simulink model "Assignment_5"  (R2025b)
settings: Solver=FixedStepAuto  StartTime=0.0  StopTime=100  FixedStep=0.05  RelTol=1e-3
settings Model: PacingRate=10  Creator=ArriGE66  LastModifiedBy=flash
settings ModelReferenceCC: EnableRefExpFcnMdlSchedulingChecks=on
settings RTWCC: GPUComputeCapability=3.5

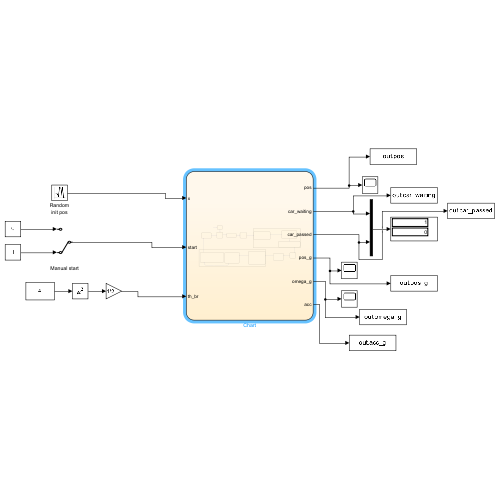
[thumbnail: Simulink's stored preview of the top-level diagram]
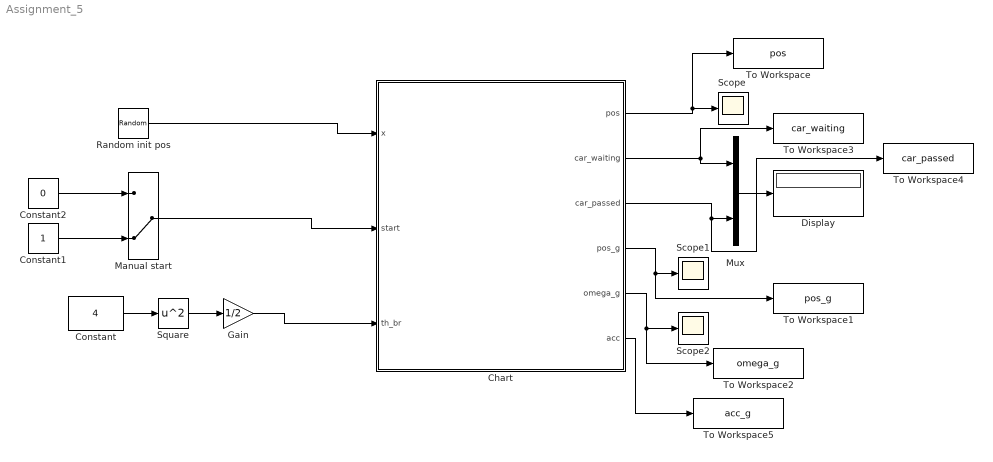
== system Assignment_5 ==
  Chart : Stateflow chart  TreatAsAtomicUnit=on
  Constant : Constant  Value=4
  Constant1 : Constant
  Constant2 : Constant  Value=0
  Display : Display
  Gain : Gain  Gain=1/2
  Manual start : ManualSwitch  CurrentSetting=0
  Mux : Mux  Inputs=2
  Random init pos : RandomNumber  Mean=-10  Variance=5
  Scope : Scope
      settings: ActiveDisplayYMinimum=-23.320975660636194  ActiveDisplayYMaximum=62.935159514485889
  Scope1 : Scope
      settings: ActiveDisplayYMinimum=-11.764436619718321  ActiveDisplayYMaximum=106.75431338028187
  Scope2 : Scope
      settings: ActiveDisplayYMinimum=-0.49999999999999989  ActiveDisplayYMaximum=4.5  DataLoggingVariableName=ScopeData2
  Square : Math  Operator=square
  To Workspace : ToWorkspace  VariableName=pos  SampleTime=-1
  To Workspace1 : ToWorkspace  VariableName=pos_g  SampleTime=-1
  To Workspace2 : ToWorkspace  VariableName=omega_g  SampleTime=-1
  To Workspace3 : ToWorkspace  VariableName=car_waiting  SampleTime=-1
  To Workspace4 : ToWorkspace  VariableName=car_passed  SampleTime=-1
  To Workspace5 : ToWorkspace  VariableName=acc_g  SampleTime=-1
  wires:
  Random init pos/1 -> Chart/1(x)
  Constant1/1 -> Manual start/2
  Constant2/1 -> Manual start/1
  Manual start/1 -> Chart/2(start)
  Chart/1(pos) -> To Workspace/1, Scope/1
  Mux/1 -> Display/1
  Chart/2(car_waiting) -> Mux/1, To Workspace3/1
  Chart/3(car_passed) -> To Workspace4/1, Mux/2
  Chart/4(pos_g) -> To Workspace1/1, Scope1/1
  Constant/1 -> Square/1
  Square/1 -> Gain/1
  Gain/1 -> Chart/3(th_br)
  Chart/5(omega_g) -> To Workspace2/1, Scope2/1
  Chart/6(acc) -> To Workspace5/1

== stateflow chart Assignment_5/Chart ==
  state INIZIO
    init_g=0;
  state RAISE FUNCTION [group]
    state RAISE_LINEAR
      acc=0;
      omega_g=omega_max;
      pos_g=init_g+omega_g*elapsed(sec);
      ex:
      pos_g=init_g+omega_g*elapsed(sec);
      init_g=pos_g;
    state RAISE_START
      acc=a;
      omega_g=acc*elapsed(sec);
      pos_g=init_g+1/2*omega_g*elapsed(sec);
      ex:
      pos_g=init_g+1/2*omega_g*elapsed(sec);
      init_g=pos_g;
    state BRAKE_RAISE
      acc=-a;
      omega_g=omega_max+acc*elapsed(sec)
      omega_g=max(0,omega_g)
      pos_g=init_g+1/2*(omega_g+omega_max)*elapsed(sec)
    RAISE_START -> RAISE_LINEAR : [omega_g>=omega_max]
    RAISE_LINEAR -> BRAKE_RAISE : [pos_g>=90-th_br]
  state IDLE
    init=x;
    pos=init;
    car_waiting=0;
    car_passed=0;
  state STOP
    tmp=pos;
    car_waiting=1;
    car_passed=0;
  state RESTART
    init_g=pos_g
    acc=0;
    pos=tmp+v*elapsed(sec);
  state APPROACHING
    pos=init+v*elapsed(sec);
  state LOWER FUNCTION [group]
    state LOWER_START
      pos=tmp+v*elapsed(sec);
      car_passed=1;
      gate_up=0;
      acc=-a;
      omega_g=acc*elapsed(sec);
      pos_g=init_g+1/2*omega_g*elapsed(sec);
      ex:
      pos_g=init_g+1/2*omega_g*elapsed(sec);
      init_g=pos_g;
      pos=tmp+v*elapsed(sec);
      tmp=pos;
    state BRAKE_LOWER
      acc=a;
      omega_g=-omega_max+acc*elapsed(sec)
      omega_g=min(0,omega_g)
      pos_g=init_g+1/2*(omega_g-omega_max)*elapsed(sec)
      pos=tmp+v*elapsed(sec);
      ex:
      pos=tmp+v*elapsed(sec);
      tmp=pos;
    state LOWER_LINEAR
      acc=0;
      omega_g=-omega_max;
      pos_g=init_g+omega_g*elapsed(sec);
      pos=tmp+v*elapsed(sec);
      ex:
      pos=tmp+v*elapsed(sec);
      tmp=pos;
      pos_g=init_g+omega_g*elapsed(sec);
      init_g=pos_g;
    LOWER_START -> LOWER_LINEAR : [omega_g<=-omega_max]
    LOWER_LINEAR -> BRAKE_LOWER : [pos_g<=0+th_br]
  state GATE_OK
    gate_up=1;
    init_g=pos_g
    acc=0;
  state PASS
    pos=tmp+v*elapsed(sec);
    car_waiting=0;
    ex:
    pos=tmp+v*elapsed(sec);
    tmp=pos;
  (default) -> INIZIO
  INIZIO -> IDLE
  IDLE -> APPROACHING : [start==1]
  RESTART -> IDLE : [after(10,sec)]
  APPROACHING -> STOP : [pos>=0]
  STOP -> RAISE_START : [car_waiting==1]
  BRAKE_LOWER -> RESTART : [omega_g==0]
  BRAKE_RAISE -> GATE_OK : [omega_g==0]
  GATE_OK -> PASS : [gate_up==1]
  PASS -> LOWER_START : [pos>= gate_end]
  data: gate_end local =5; v local double =1; pos output; car_waiting output; car_passed output; init local; x input; start input; tmp local; a local =1; pos_g output; gate_up local; init_g local; omega_max local =4; th_br input; omega_g output; acc output
